simulink model "step4"  (R2021a)
settings: Solver=FixedStepAuto  StartTime=0.0  StopTime=2000  FixedStep=0.001  RelTol=1e-3
settings Model: Creator=konsta  LastModifiedBy=konsta

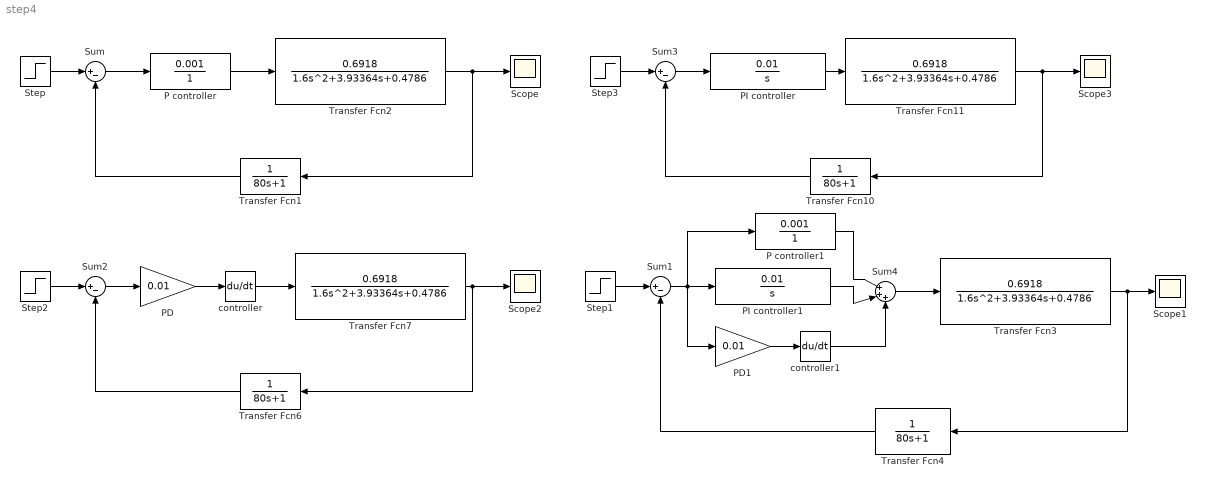
== system step4 ==
  P controller : TransferFcn  Numerator=[0.001]  Denominator=[0 1]
  P controller1 : TransferFcn  Numerator=[0.001]  Denominator=[0 1]
  PD : Gain  Gain=0.01
  PD1 : Gain  Gain=0.01
  PI controller : TransferFcn  Numerator=[0.01]  Denominator=[1 0 ]
  PI controller1 : TransferFcn  Numerator=[0.01]  Denominator=[1 0 ]
  Scope{,1..3} (4 alike) : Scope
  Step{,1..3} (4 alike) : Step  SampleTime=0
  Sum{,1..3} (4 alike) : Sum  Inputs=|+-
  Sum4 : Sum  Inputs=|+++
  Transfer Fcn{1,4,6,10} (4 alike) : TransferFcn  Denominator=[80 1]
  Transfer Fcn{2..3,7,11} (4 alike) : TransferFcn  Numerator=[0.6918]  Denominator=[1.6 3.93364 0.4786]
  controller : Derivative
  controller1 : Derivative
  wires:
  P controller/1 -> Transfer Fcn2/1
  Transfer Fcn2/1 -> Transfer Fcn1/1, Scope/1
  Transfer Fcn1/1 -> Sum/2
  Sum/1 -> P controller/1
  Step/1 -> Sum/1
  Transfer Fcn10/1 -> Sum3/2
  Step3/1 -> Sum3/1
  Sum3/1 -> PI controller/1
  Transfer Fcn11/1 -> Transfer Fcn10/1, Scope3/1
  PI controller/1 -> Transfer Fcn11/1
  Step2/1 -> Sum2/1
  Transfer Fcn7/1 -> Transfer Fcn6/1, Scope2/1
  Transfer Fcn6/1 -> Sum2/2
  Transfer Fcn4/1 -> Sum1/2
  Step1/1 -> Sum1/1
  Transfer Fcn3/1 -> Transfer Fcn4/1, Scope1/1
  Sum4/1 -> Transfer Fcn3/1
  Sum1/1 -> PD1/1, P controller1/1, PI controller1/1
  P controller1/1 -> Sum4/1
  PI controller1/1 -> Sum4/2
  PD/1 -> controller/1
  controller/1 -> Transfer Fcn7/1
  Sum2/1 -> PD/1
  PD1/1 -> controller1/1
  controller1/1 -> Sum4/3
